simulink model "lab7_3"  (R2018b)
settings: Solver=FixedStepDiscrete  StartTime=0.0  StopTime=1000  FixedStep=1  RelTol=1e-3
libraries: hdlsllib x2, simulink x1
settings Model: Creator=mllax8  LastModifiedBy=mllax8

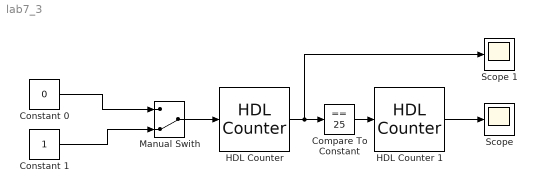
== system lab7_3 ==
  Compare To Constant : simulink/Logic and Bit Operations/Compare To Constant  relop===  const=25  OutDataTypeStr=boolean
  Constant 0 : Constant  Value=0  OutDataTypeStr=boolean
  Constant 1 : Constant  OutDataTypeStr=boolean
  "HDL Counter " : hdlsllib/Sources/HDL Counter  CountType=Free running  CountInit=0  CountStep=1  CountMax=25  CountFromType=Initial value  CountFrom=0  CountResetPort=off  CountLoadPort=off  CountEnbPort=on  CountDirPort=off  CountDataType=Unsigned  CountWordLen=8  CountFracLen=0  CountSampTime=1
      settings: SourceProductBaseCode=HD
  HDL Counter 1 : hdlsllib/Sources/HDL Counter  CountType=Free running  CountInit=0  CountStep=1  CountMax=25  CountFromType=Initial value  CountFrom=0  CountResetPort=off  CountLoadPort=off  CountEnbPort=on  CountDirPort=off  CountDataType=Unsigned  CountWordLen=8  CountFracLen=0  CountSampTime=1
      settings: SourceProductBaseCode=HD
  Manual Swith : ManualSwitch  CurrentSetting=0
  "Scope " : Scope
  Scope 1 : Scope
  wires:
  Constant 0/1 -> Manual Swith/1
  Constant 1/1 -> Manual Swith/2
  Manual Swith/1 -> "HDL Counter "/1
  "HDL Counter "/1 -> Scope 1/1, Compare To Constant/1
  Compare To Constant/1 -> HDL Counter 1/1
  HDL Counter 1/1 -> "Scope "/1
